simulink model "Lab1_Analog_Control_System_Design"  (R2014a)
settings: Solver=ode23t  StartTime=0.0  StopTime=20  RelTol=1e-3
settings Model: Creator=cloughj  LastModifiedBy=cloughj

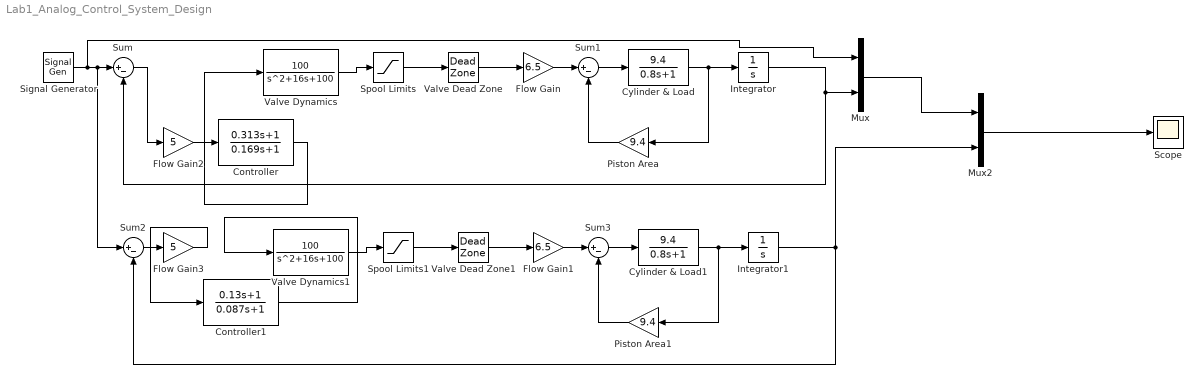
== system Lab1_Analog_Control_System_Design ==
  Controller : TransferFcn  Numerator=[0.313 1]  Denominator=[0.169 1]
  Controller1 : TransferFcn  Numerator=[0.13 1]  Denominator=[0.087 1]
  Cylinder & Load : TransferFcn  Numerator=[9.4]  Denominator=[0.8 1]
  Cylinder & Load1 : TransferFcn  Numerator=[9.4]  Denominator=[0.8 1]
  Flow Gain : Gain  Gain=6.5
  Flow Gain1 : Gain  Gain=6.5
  Flow Gain2 : Gain  Gain=5
  Flow Gain3 : Gain  Gain=5
  Integrator : Integrator
  Integrator1 : Integrator
  Mux : Mux  Inputs=2
  Mux2 : Mux  Inputs=2
  Piston Area : Gain  Gain=9.4
  Piston Area1 : Gain  Gain=9.4
  Scope : Scope
  Signal Generator : SignalGenerator  WaveForm=square  Frequency=0.1
  Spool Limits : Saturate  UpperLimit=inf  LowerLimit=-inf
  Spool Limits1 : Saturate  UpperLimit=inf  LowerLimit=-inf
  Sum{,1..3} (4 alike) : Sum  Inputs=|+-
  Valve Dead Zone : DeadZone  LowerValue=0  UpperValue=0  SaturateOnIntegerOverflow=on
  Valve Dead Zone1 : DeadZone  LowerValue=0  UpperValue=0  SaturateOnIntegerOverflow=on
  Valve Dynamics : TransferFcn  Numerator=[100]  Denominator=[1 16 100]
  Valve Dynamics1 : TransferFcn  Numerator=[100]  Denominator=[1 16 100]
  wires:
  Controller/1 -> Valve Dynamics/1
  Valve Dynamics/1 -> Spool Limits/1
  Valve Dead Zone/1 -> Flow Gain/1
  Flow Gain/1 -> Sum1/1
  Sum1/1 -> Cylinder & Load/1
  Cylinder & Load/1 -> Piston Area/1, Integrator/1
  Integrator/1 -> Sum/2, Mux/2
  Piston Area/1 -> Sum1/2
  Spool Limits/1 -> Valve Dead Zone/1
  Valve Dynamics1/1 -> Spool Limits1/1
  Valve Dead Zone1/1 -> Flow Gain1/1
  Flow Gain1/1 -> Sum3/1
  Sum3/1 -> Cylinder & Load1/1
  Cylinder & Load1/1 -> Piston Area1/1, Integrator1/1
  Integrator1/1 -> Mux2/2, Sum2/2
  Signal Generator/1 -> Sum2/1, Sum/1, Mux/1
  Piston Area1/1 -> Sum3/2
  Spool Limits1/1 -> Valve Dead Zone1/1
  Mux/1 -> Mux2/1
  Mux2/1 -> Scope/1
  Flow Gain2/1 -> Controller/1
  Sum/1 -> Flow Gain2/1
  Sum2/1 -> Flow Gain3/1
  Flow Gain3/1 -> Controller1/1
  Controller1/1 -> Valve Dynamics1/1
